simulink model "Microgrid_w_BESS"  (R2024b)
settings: Solver=VariableStepAuto  StartTime=0.0  StopTime=4  RelTol=1e-3
undefined symbols (not defined in the file or in its folder): Ion, Lithium, Ts_Control
libraries: spsParallelRLCBranchLib x8, simulink x6, spsSeriesRLCBranchLib x6, powerlib_extras x6, ee_lib x5, nesl_utility x5, slpidlib x5, spsThreePhaseVIMeasurementLib x3, spsThreePhaseSeriesRLCBranchLib x3, spsCurrentVoltageSimscapeInterfaceLib x3, eePowerMeasurement x3, spsVoltageMeasurementLib x2
(part 2 of 2)

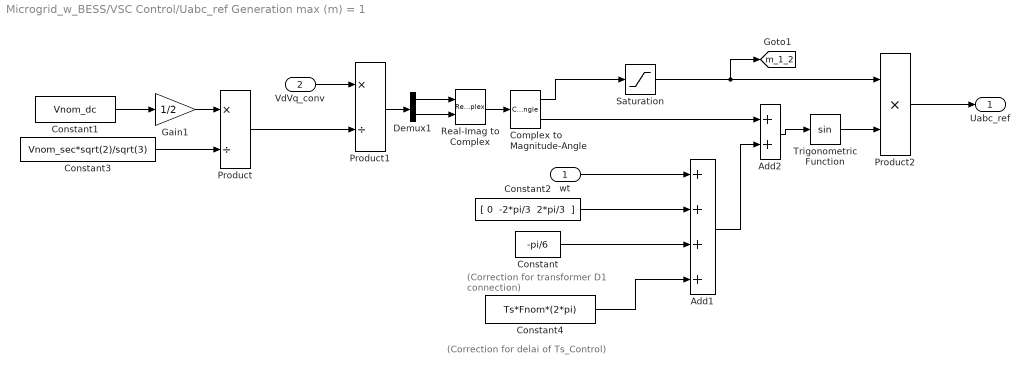
== system Microgrid_w_BESS/VSC Control/Uabc_ref Generation max (m) = 1 ==
  note: (Correction for delai of Ts_Control)
  note: (Correction for transformer
      |  D1 connection)
  wt : Inport
  VdVq_conv : Inport  Port=2
  Add1 : Sum  Inputs=++++
  Add2 : Sum
  Complex to Magnitude-Angle : ComplexToMagnitudeAngle
  Constant : Constant  Value=-pi/6
  Constant1 : Constant  Value=Vnom_dc
  Constant2 : Constant  Value="[ 0  -2*pi/3  2*pi/3  ]"
  Constant3 : Constant  Value=Vnom_sec*sqrt(2)/sqrt(3)
  Constant4 : Constant  Value=Ts*Fnom*(2*pi)
  Demux1 : Demux  Outputs=2
  Gain1 : Gain  Gain=1/2
  Product : Product  Inputs=*/  RndMeth=Zero
  Product1 : Product  Inputs=*/  RndMeth=Zero
  Product2 : Product  Inputs=**  RndMeth=Zero
  Real-Imag to Complex : RealImagToComplex
  Saturation : Saturate  UpperLimit=1  LowerLimit=0
  Trigonometric Function : Trigonometry
  Uabc_ref : Outport  VectorParamsAs1DForOutWhenUnconnected=off
  tag scope: m_1_2=global
  wires:
  Constant4/1 -> Add1/4
  wt/1 -> Add1/1
  Product2/1 -> Uabc_ref/1
  Trigonometric Function/1 -> Product2/2
  Saturation/1 -> Product2/1, [m_1_2]
  Add2/1 -> Trigonometric Function/1
  Add1/1 -> Add2/2
  Complex to Magnitude-Angle/2 -> Add2/1
  Product/1 -> Product1/2
  Constant3/1 -> Product/2
  Constant/1 -> Add1/3
  Constant2/1 -> Add1/2
  Demux1/2 -> Real-Imag to Complex/2
  Demux1/1 -> Real-Imag to Complex/1
  Real-Imag to Complex/1 -> Complex to Magnitude-Angle/1
  Gain1/1 -> Product/1
  Product1/1 -> Demux1/1
  VdVq_conv/1 -> Product1/1
  Constant1/1 -> Gain1/1
  Complex to Magnitude-Angle/1 -> Saturation/1

== system Microgrid_w_BESS/VSC Control/VDC Regulator ==
  Vdc_meas : Inport  PortDimensions=1
  Vdc_ref : Inport  Port=2  PortDimensions=1
  PI : slpidlib/PID Controller  Controller=PI  Form=Parallel  TimeDomain=Discrete-time  UseExternalTs=off  SampleTime=Ts  IntegratorMethod=Trapezoidal  FilterMethod=Forward Euler  ControllerParametersSource=internal  P=Kp_VDCreg  I=Ki_VDCreg  UseKiTs=off  D=0  UseExternalDerivativeSource=off  N=100  UseFilter=on  TunerSelectOption=Transfer Function Based (PID Tuner App)  InitialConditionSource=internal  InitialConditionForIntegrator=0  InitialConditionForFilter=0  DifferentiatorICPrevScaledInput=0  ExternalReset=none  TrackingMode=off  Kt=1  LimitOutput=on  SatLimitsSource=internal  UpperSaturationLimit=1.5  LowerSaturationLimit=-1.5  LinearizeAsGain=off  AntiWindupMode=none  Kb=1  LimitIntegrator=off  UpperIntegratorSaturationLimit=inf  LowerIntegratorSaturationLimit=-inf  POutMin=[]  POutMax=[]  IOutMin=[]  IOutMax=[]  DOutMin=[]  DOutMax=[]  NOutMin=[]  NOutMax=[]  SumOutMin=[]  SumOutMax=[]  SaturationOutMin=[]  SaturationOutMax=[]  PParamMin=[]  PParamMax=[]  IParamMin=[]  IParamMax=[]  DParamMin=[]  DParamMax=[]  NParamMin=[]  NParamMax=[]  KbParamMin=[]  KbParamMax=[]  KtParamMin=[]  KtParamMax=[]  KbOutMin=[]  KbOutMax=[]  KtOutMin=[]  KtOutMax=[]  IntegratorOutMin=[]  IntegratorOutMax=[]  FilterOutMin=[]  FilterOutMax=[]  SumI1OutMin=[]  SumI1OutMax=[]  SumI2OutMin=[]  SumI2OutMax=[]  SumI3OutMin=[]  SumI3OutMax=[]  SumI4OutMin=[]  SumI4OutMax=[]  SumDOutMin=[]  SumDOutMax=[]  DifferentiatorOutMin=[]  DifferentiatorOutMax=[]  FilterDiffOutCoefMin=[]  FilterDiffOutCoefMax=[]  ReciprocalOutMin=[]  ReciprocalOutMax=[]  SumDenOutMin=[]  SumDenOutMax=[]  SumNumOutMin=[]  SumNumOutMax=[]  DivideOutMin=[]  DivideOutMax=[]  UdiffTsProdOutMin=[]  UdiffTsProdOutMax=[]  NTsProdOutMin=[]  NTsProdOutMax=[]  UintegralTsProdOutMin=[]  UintegralTsProdOutMax=[]  UngainTsProdOutMin=[]  UngainTsProdOutMax=[]  ClampingZeroOutDataTypeStr=Inherit: Inherit via back propagation  ClampingZeroOutMin=[]  ClampingZeroOutMax=[]  FilterDenConstantOutDataTypeStr=Inherit: Inherit via back propagation  FilterDenConstantOutMin=[]  FilterDenConstantOutMax=[]  PCopyOutDataTypeStr=Inherit: Inherit via back propagation  PCopyOutMin=[]  PCopyOutMax=[]  NCopyOutDataTypeStr=Inherit: Inherit via back propagation  NCopyOutMin=[]  NCopyOutMax=[]  IntegratorContinuousStateAttributes=''  IntegratorStateMustResolveToSignalObject=off  IntegratorRTWStateStorageClass=Auto  FilterContinuousStateAttributes=''  FilterStateMustResolveToSignalObject=off  FilterRTWStateStorageClass=Auto  ParallelPVariant=InternalParameters  IdealPVariant=Disabled  IVariant=InternalParameters  DVariant=Disabled  IntegratorVariant=Discrete  SatVariant=Enabled  AWVariant=Passthrough  PCopyVariant=Disabled  TRVariant=Disabled  FdbkBlocksVariant=Forward  IdealPFdbkVariant=Disabled  SatFdbkVariant=Disabled  DerivativeFilterVariant=Disabled  NVariant=Disabled  NCopyVariant=Disabled_SignalSpec  FilterICVariant=Disabled  IntegratorICVariant=InternalICs  ExternalResetVariant=Disabled  TRSumVariant=Passthrough  SumFdbkVariant=Disabled  SumVariant=Sum_PI  TsampFilterVariant=InternalTs  TsampNgainVariant=Passthrough  TsampIntegralVariant=Disabled_SignalSpec  ExternalSaturationOutDataTypeStr=Inherit: Same as second input  DerivativeSourceVariant=Disabled  PreIntVariant=InternalPreInt
  Rtot_pu3 : Gain  Gain=1/Vnom_dc  SaturateOnIntegerOverflow=on  OutDataTypeStr=Inherit: Same as input  ParamDataTypeStr=Inherit: Same as input
  Sum : Sum  Inputs=|+-
  Id_ref : Outport  SampleTime=Ts  InitialOutput=0  VectorParamsAs1DForOutWhenUnconnected=off
  tag scope: Id_ref_2=global, Vdc_ref_2=global
  wires:
  Rtot_pu3/1 -> PI/1
  Vdc_ref/1 -> [Vdc_ref_2], Sum/2
  Vdc_meas/1 -> Sum/1
  Sum/1 -> Rtot_pu3/1
  PI/1 -> [Id_ref_2], Id_ref/1

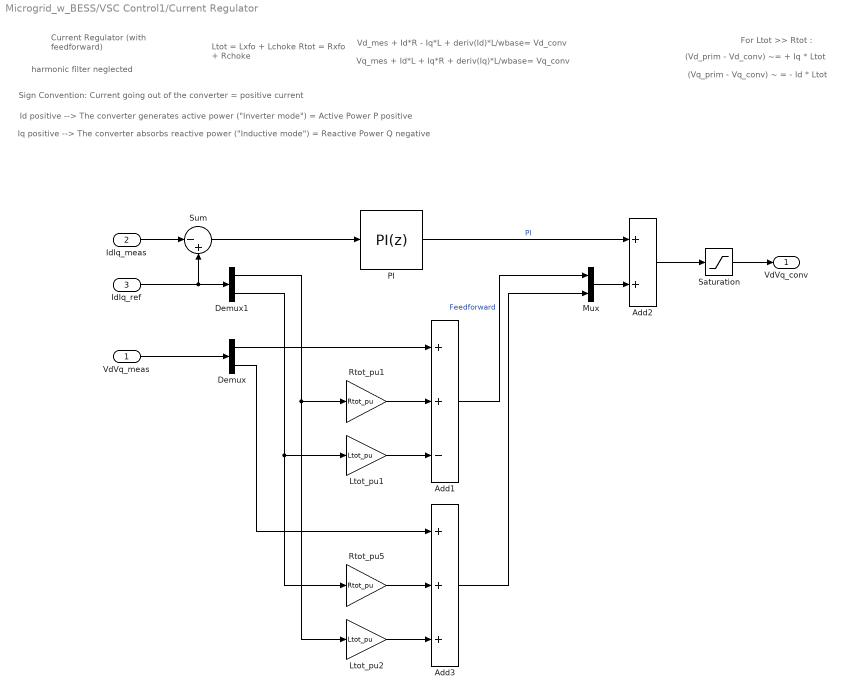
== system Microgrid_w_BESS/VSC Control1/Current Regulator ==
  note: harmonic filter neglected
  note: Vd_mes + Id*R - Iq*L + deriv(Id)*L/wbase= Vd_conv
  note: Vq_mes + Id*L + Iq*R + deriv(Iq)*L/wbase= Vq_conv
  note: Current Regulator
      | (with feedforward)
  note: Sign Convention: Current going out of the converter = positive current
  note: Iq positive --> The converter absorbs reactive power ("Inductive mode") = Reactive Power Q negative
  note: Id positive --> The converter generates active power ("Inverter mode") = Active Power P positive
  note: Ltot = Lxfo + Lchoke
      | Rtot = Rxfo + Rchoke
  note: (Vd_prim - Vd_conv) ~= + Iq * Ltot
  note: (Vq_prim - Vq_conv) ~ = - Id * Ltot
  note: For Ltot >> Rtot :
  VdVq_meas : Inport  PortDimensions=2
  IdIq_meas : Inport  Port=2  PortDimensions=2
  IdIq_ref : Inport  Port=3  PortDimensions=2
  Add1 : Sum  Inputs=++-
  Add2 : Sum
  Add3 : Sum  Inputs=+++
  Demux : Demux  Outputs=2
  Demux1 : Demux  Outputs=2
  Ltot_pu1 : Gain  Gain=Ltot_pu  SaturateOnIntegerOverflow=on  OutDataTypeStr=Inherit: Same as input  ParamDataTypeStr=Inherit: Same as input
  Ltot_pu2 : Gain  Gain=Ltot_pu  SaturateOnIntegerOverflow=on  OutDataTypeStr=Inherit: Same as input  ParamDataTypeStr=Inherit: Same as input
  Mux : Mux  Inputs=2
  PI : slpidlib/PID Controller  Controller=PI  Form=Parallel  TimeDomain=Discrete-time  UseExternalTs=off  SampleTime=Ts  IntegratorMethod=Forward Euler  FilterMethod=Forward Euler  ControllerParametersSource=internal  P=Kp_Ireg  I=Ki_Ireg  UseKiTs=off  D=0  UseExternalDerivativeSource=off  N=100  UseFilter=on  TunerSelectOption=Transfer Function Based (PID Tuner App)  InitialConditionSource=internal  InitialConditionForIntegrator=0  InitialConditionForFilter=0  DifferentiatorICPrevScaledInput=0  ExternalReset=none  TrackingMode=off  Kt=1  LimitOutput=on  SatLimitsSource=internal  UpperSaturationLimit=2  LowerSaturationLimit=-2  LinearizeAsGain=off  AntiWindupMode=none  Kb=1  LimitIntegrator=off  UpperIntegratorSaturationLimit=inf  LowerIntegratorSaturationLimit=-inf  POutMin=[]  POutMax=[]  IOutMin=[]  IOutMax=[]  DOutMin=[]  DOutMax=[]  NOutMin=[]  NOutMax=[]  SumOutMin=[]  SumOutMax=[]  SaturationOutMin=[]  SaturationOutMax=[]  PParamMin=[]  PParamMax=[]  IParamMin=[]  IParamMax=[]  DParamMin=[]  DParamMax=[]  NParamMin=[]  NParamMax=[]  KbParamMin=[]  KbParamMax=[]  KtParamMin=[]  KtParamMax=[]  KbOutMin=[]  KbOutMax=[]  KtOutMin=[]  KtOutMax=[]  IntegratorOutMin=[]  IntegratorOutMax=[]  FilterOutMin=[]  FilterOutMax=[]  SumI1OutMin=[]  SumI1OutMax=[]  SumI2OutMin=[]  SumI2OutMax=[]  SumI3OutMin=[]  SumI3OutMax=[]  SumI4OutMin=[]  SumI4OutMax=[]  SumDOutMin=[]  SumDOutMax=[]  DifferentiatorOutMin=[]  DifferentiatorOutMax=[]  FilterDiffOutCoefMin=[]  FilterDiffOutCoefMax=[]  ReciprocalOutMin=[]  ReciprocalOutMax=[]  SumDenOutMin=[]  SumDenOutMax=[]  SumNumOutMin=[]  SumNumOutMax=[]  DivideOutMin=[]  DivideOutMax=[]  UdiffTsProdOutMin=[]  UdiffTsProdOutMax=[]  NTsProdOutMin=[]  NTsProdOutMax=[]  UintegralTsProdOutMin=[]  UintegralTsProdOutMax=[]  UngainTsProdOutMin=[]  UngainTsProdOutMax=[]  ClampingZeroOutDataTypeStr=Inherit: Inherit via back propagation  ClampingZeroOutMin=[]  ClampingZeroOutMax=[]  FilterDenConstantOutDataTypeStr=Inherit: Inherit via back propagation  FilterDenConstantOutMin=[]  FilterDenConstantOutMax=[]  PCopyOutDataTypeStr=Inherit: Inherit via back propagation  PCopyOutMin=[]  PCopyOutMax=[]  NCopyOutDataTypeStr=Inherit: Inherit via back propagation  NCopyOutMin=[]  NCopyOutMax=[]  IntegratorContinuousStateAttributes=''  IntegratorStateMustResolveToSignalObject=off  IntegratorRTWStateStorageClass=Auto  FilterContinuousStateAttributes=''  FilterStateMustResolveToSignalObject=off  FilterRTWStateStorageClass=Auto  ParallelPVariant=InternalParameters  IdealPVariant=Disabled  IVariant=InternalParameters  DVariant=Disabled  IntegratorVariant=Discrete  SatVariant=Enabled  AWVariant=Passthrough  PCopyVariant=Disabled  TRVariant=Disabled  FdbkBlocksVariant=Forward  IdealPFdbkVariant=Disabled  SatFdbkVariant=Disabled  DerivativeFilterVariant=Disabled  NVariant=Disabled  NCopyVariant=Disabled_SignalSpec  FilterICVariant=Disabled  IntegratorICVariant=InternalICs  ExternalResetVariant=Disabled  TRSumVariant=Passthrough  SumFdbkVariant=Disabled  SumVariant=Sum_PI  TsampFilterVariant=InternalTs  TsampNgainVariant=Passthrough  TsampIntegralVariant=Disabled_SignalSpec  ExternalSaturationOutDataTypeStr=Inherit: Same as second input  DerivativeSourceVariant=Disabled  PreIntVariant=InternalPreInt
  Rtot_pu1 : Gain  Gain=Rtot_pu  SaturateOnIntegerOverflow=on  OutDataTypeStr=Inherit: Same as input  ParamDataTypeStr=Inherit: Same as input
  Rtot_pu5 : Gain  Gain=Rtot_pu  SaturateOnIntegerOverflow=on  OutDataTypeStr=Inherit: Same as input  ParamDataTypeStr=Inherit: Same as input
  Saturation : Saturate  UpperLimit=2  LowerLimit=-2
  Sum : Sum  Inputs=|-+
  VdVq_conv : Outport  VectorParamsAs1DForOutWhenUnconnected=off
  wires:
  Mux/1 -> Add2/2
  PI/1 -> Add2/1  "PI"
  Sum/1 -> PI/1
  IdIq_ref/1 -> Sum/2, Demux1/1
  IdIq_meas/1 -> Sum/1
  Add2/1 -> Saturation/1
  Saturation/1 -> VdVq_conv/1
  VdVq_meas/1 -> Demux/1
  Demux/1 -> Add1/1
  Rtot_pu1/1 -> Add1/2
  Demux1/1 -> Rtot_pu1/1, Ltot_pu2/1
  Ltot_pu1/1 -> Add1/3
  Demux1/2 -> Ltot_pu1/1, Rtot_pu5/1
  Rtot_pu5/1 -> Add3/2
  Ltot_pu2/1 -> Add3/3
  Add1/1 -> Mux/1  "Feedforward"
  Demux/2 -> Add3/1
  Add3/1 -> Mux/2

== system Microgrid_w_BESS/VSC Control1/Inverter ON//OFF Logic ==
  V_DC : Inport
  AND : Logic  Operator=NAND  IconShape=distinctive  AllPortsSameDT=off  OutDataTypeStr=boolean
  Compare To Constant : simulink/Logic and Bit Operations/Compare To Constant  relop=>=  const=200  OutDataTypeStr=boolean
  Constant : Constant
  Data Type Conversion : DataTypeConversion  OutDataTypeStr=double  SaturateOnIntegerOverflow=off  RndMeth=Floor
  BL : Outport
  tag scope: inv_cont_1=global
  wires:
  Constant/1 -> AND/2
  Compare To Constant/1 -> AND/1
  AND/1 -> Data Type Conversion/1
  V_DC/1 -> Compare To Constant/1
  Data Type Conversion/1 -> BL/1, [inv_cont_1]

== system Microgrid_w_BESS/VSC Control1/PLL & Measurements ==
  Vabc_prim : Inport
  Iabc_prim : Inport  Port=2
  PLL : powerlib_extras/Discrete  Control Blocks/Discrete 3-phase PLL  Fmin=45  Par_Init="[-0.57  Fnom]"  ParK=[60 1400]  Ts=Ts  AGC=off
  Selector1 : Selector  InputPortWidth=3  IndexOptions=Index vector (dialog)  Indices=[1 2]  OutputSizes=1
  Selector2 : Selector  InputPortWidth=3  IndexOptions=Index vector (dialog)  Indices=[1 2]  OutputSizes=1
  Terminator : Terminator
  V->pu : Gain  Gain=1/(Vnom_prim*sqrt(2)/sqrt(3))  SaturateOnIntegerOverflow=on  OutDataTypeStr=Inherit: Same as input  ParamDataTypeStr=Inherit: Same as input
  V->pu1 : Gain  Gain=Vnom_prim*sqrt(3)/Pnom/sqrt(2)  SaturateOnIntegerOverflow=on  OutDataTypeStr=Inherit: Same as input  ParamDataTypeStr=Inherit: Same as input
  abc_to_dq0 Transformation1 : powerlib_extras/Measurements/abc_to_dq0 Transformation
  abc_to_dq0 Transformation2 : powerlib_extras/Measurements/abc_to_dq0 Transformation
  wt : Outport  VectorParamsAs1DForOutWhenUnconnected=off
  VdVq_prim : Outport  Port=2  VectorParamsAs1DForOutWhenUnconnected=off
  IdIq_prim : Outport  Port=3  VectorParamsAs1DForOutWhenUnconnected=off
  wires:
  V->pu1/1 -> abc_to_dq0 Transformation2/1
  V->pu/1 -> PLL/1, abc_to_dq0 Transformation1/1
  abc_to_dq0 Transformation2/1 -> Selector1/1
  PLL/2 -> wt/1
  Vabc_prim/1 -> V->pu/1
  Iabc_prim/1 -> V->pu1/1
  abc_to_dq0 Transformation1/1 -> Selector2/1
  Selector2/1 -> VdVq_prim/1
  Selector1/1 -> IdIq_prim/1
  PLL/3 -> abc_to_dq0 Transformation2/2, abc_to_dq0 Transformation1/2
  PLL/1 -> Terminator/1

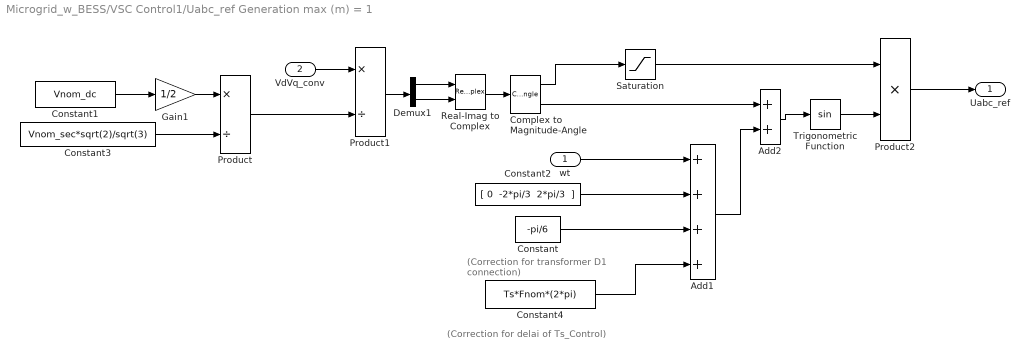
== system Microgrid_w_BESS/VSC Control1/Uabc_ref Generation max (m) = 1 ==
  note: (Correction for transformer
      |  D1 connection)
  note: (Correction for delai of Ts_Control)
  wt : Inport
  VdVq_conv : Inport  Port=2
  Add1 : Sum  Inputs=++++
  Add2 : Sum
  Complex to Magnitude-Angle : ComplexToMagnitudeAngle
  Constant : Constant  Value=-pi/6
  Constant1 : Constant  Value=Vnom_dc
  Constant2 : Constant  Value="[ 0  -2*pi/3  2*pi/3  ]"
  Constant3 : Constant  Value=Vnom_sec*sqrt(2)/sqrt(3)
  Constant4 : Constant  Value=Ts*Fnom*(2*pi)
  Demux1 : Demux  Outputs=2
  Gain1 : Gain  Gain=1/2
  Product : Product  Inputs=*/  RndMeth=Zero
  Product1 : Product  Inputs=*/  RndMeth=Zero
  Product2 : Product  Inputs=**  RndMeth=Zero
  Real-Imag to Complex : RealImagToComplex
  Saturation : Saturate  UpperLimit=1  LowerLimit=0
  Trigonometric Function : Trigonometry
  Uabc_ref : Outport  VectorParamsAs1DForOutWhenUnconnected=off
  wires:
  Complex to Magnitude-Angle/1 -> Saturation/1
  Constant1/1 -> Gain1/1
  VdVq_conv/1 -> Product1/1
  Product1/1 -> Demux1/1
  Gain1/1 -> Product/1
  Real-Imag to Complex/1 -> Complex to Magnitude-Angle/1
  Demux1/1 -> Real-Imag to Complex/1
  Demux1/2 -> Real-Imag to Complex/2
  Constant2/1 -> Add1/2
  Constant/1 -> Add1/3
  Constant3/1 -> Product/2
  Product/1 -> Product1/2
  Complex to Magnitude-Angle/2 -> Add2/1
  Add1/1 -> Add2/2
  Add2/1 -> Trigonometric Function/1
  Saturation/1 -> Product2/1
  Trigonometric Function/1 -> Product2/2
  Product2/1 -> Uabc_ref/1
  wt/1 -> Add1/1
  Constant4/1 -> Add1/4

== system Microgrid_w_BESS/VSC Control1/VDC Regulator ==
  Vdc_meas : Inport  PortDimensions=1
  Vdc_ref : Inport  Port=2  PortDimensions=1
  PI : slpidlib/PID Controller  Controller=PI  Form=Parallel  TimeDomain=Discrete-time  UseExternalTs=off  SampleTime=Ts  IntegratorMethod=Trapezoidal  FilterMethod=Forward Euler  ControllerParametersSource=internal  P=Kp_VDCreg  I=Ki_VDCreg  UseKiTs=off  D=0  UseExternalDerivativeSource=off  N=100  UseFilter=on  TunerSelectOption=Transfer Function Based (PID Tuner App)  InitialConditionSource=internal  InitialConditionForIntegrator=0  InitialConditionForFilter=0  DifferentiatorICPrevScaledInput=0  ExternalReset=none  TrackingMode=off  Kt=1  LimitOutput=on  SatLimitsSource=internal  UpperSaturationLimit=1.5  LowerSaturationLimit=-1.5  LinearizeAsGain=off  AntiWindupMode=none  Kb=1  LimitIntegrator=off  UpperIntegratorSaturationLimit=inf  LowerIntegratorSaturationLimit=-inf  POutMin=[]  POutMax=[]  IOutMin=[]  IOutMax=[]  DOutMin=[]  DOutMax=[]  NOutMin=[]  NOutMax=[]  SumOutMin=[]  SumOutMax=[]  SaturationOutMin=[]  SaturationOutMax=[]  PParamMin=[]  PParamMax=[]  IParamMin=[]  IParamMax=[]  DParamMin=[]  DParamMax=[]  NParamMin=[]  NParamMax=[]  KbParamMin=[]  KbParamMax=[]  KtParamMin=[]  KtParamMax=[]  KbOutMin=[]  KbOutMax=[]  KtOutMin=[]  KtOutMax=[]  IntegratorOutMin=[]  IntegratorOutMax=[]  FilterOutMin=[]  FilterOutMax=[]  SumI1OutMin=[]  SumI1OutMax=[]  SumI2OutMin=[]  SumI2OutMax=[]  SumI3OutMin=[]  SumI3OutMax=[]  SumI4OutMin=[]  SumI4OutMax=[]  SumDOutMin=[]  SumDOutMax=[]  DifferentiatorOutMin=[]  DifferentiatorOutMax=[]  FilterDiffOutCoefMin=[]  FilterDiffOutCoefMax=[]  ReciprocalOutMin=[]  ReciprocalOutMax=[]  SumDenOutMin=[]  SumDenOutMax=[]  SumNumOutMin=[]  SumNumOutMax=[]  DivideOutMin=[]  DivideOutMax=[]  UdiffTsProdOutMin=[]  UdiffTsProdOutMax=[]  NTsProdOutMin=[]  NTsProdOutMax=[]  UintegralTsProdOutMin=[]  UintegralTsProdOutMax=[]  UngainTsProdOutMin=[]  UngainTsProdOutMax=[]  ClampingZeroOutDataTypeStr=Inherit: Inherit via back propagation  ClampingZeroOutMin=[]  ClampingZeroOutMax=[]  FilterDenConstantOutDataTypeStr=Inherit: Inherit via back propagation  FilterDenConstantOutMin=[]  FilterDenConstantOutMax=[]  PCopyOutDataTypeStr=Inherit: Inherit via back propagation  PCopyOutMin=[]  PCopyOutMax=[]  NCopyOutDataTypeStr=Inherit: Inherit via back propagation  NCopyOutMin=[]  NCopyOutMax=[]  IntegratorContinuousStateAttributes=''  IntegratorStateMustResolveToSignalObject=off  IntegratorRTWStateStorageClass=Auto  FilterContinuousStateAttributes=''  FilterStateMustResolveToSignalObject=off  FilterRTWStateStorageClass=Auto  ParallelPVariant=InternalParameters  IdealPVariant=Disabled  IVariant=InternalParameters  DVariant=Disabled  IntegratorVariant=Discrete  SatVariant=Enabled  AWVariant=Passthrough  PCopyVariant=Disabled  TRVariant=Disabled  FdbkBlocksVariant=Forward  IdealPFdbkVariant=Disabled  SatFdbkVariant=Disabled  DerivativeFilterVariant=Disabled  NVariant=Disabled  NCopyVariant=Disabled_SignalSpec  FilterICVariant=Disabled  IntegratorICVariant=InternalICs  ExternalResetVariant=Disabled  TRSumVariant=Passthrough  SumFdbkVariant=Disabled  SumVariant=Sum_PI  TsampFilterVariant=InternalTs  TsampNgainVariant=Passthrough  TsampIntegralVariant=Disabled_SignalSpec  ExternalSaturationOutDataTypeStr=Inherit: Same as second input  DerivativeSourceVariant=Disabled  PreIntVariant=InternalPreInt
  Rtot_pu3 : Gain  Gain=1/Vnom_dc  SaturateOnIntegerOverflow=on  OutDataTypeStr=Inherit: Same as input  ParamDataTypeStr=Inherit: Same as input
  Sum : Sum  Inputs=|+-
  Id_ref : Outport  SampleTime=Ts  InitialOutput=0  VectorParamsAs1DForOutWhenUnconnected=off
  wires:
  PI/1 -> Id_ref/1
  Sum/1 -> Rtot_pu3/1
  Vdc_meas/1 -> Sum/1
  Vdc_ref/1 -> Sum/2
  Rtot_pu3/1 -> PI/1

== system Microgrid_w_BESS/BESS/BATT chg-dshg logic1/Unused ==
  Charging : Constant  Commented=on
  MATLAB Function : MATLAB Function  Commented=on  TreatAsAtomicUnit=on
  MATLAB Function1 : MATLAB Function  Commented=on  TreatAsAtomicUnit=on
  MATLAB Function2 : MATLAB Function  Commented=on  TreatAsAtomicUnit=on
  MATLAB Function7 : MATLAB Function  Commented=on  TreatAsAtomicUnit=on
  MATLAB Function8 : MATLAB Function  Commented=on  TreatAsAtomicUnit=on
  Manual Switch : ManualSwitch  Commented=on  CurrentSetting=0
  discharging : Constant  Commented=on  Value=0
  Out1 : Outport
  wires:
  Manual Switch/1 -> Out1/1
  Charging/1 -> Manual Switch/2
  discharging/1 -> Manual Switch/1

== matlab function Microgrid_w_BESS/BESS/BATT chg-dshg logic1/Unused/MATLAB Function7 ==
  data: Vdc input; D output; Vbatt input; I_batt_meas input; I_batt_ref_mag input; Ts input
function D = controller_discharging(Vdc, Vbatt, I_batt_meas, I_batt_ref_mag, Ts)
%#codegen
% Limits
Imax_discharge = -50;
% PI gains for discharging (tuned for damping)
Kp = 0.3; % Increased for quicker response
Ki = 0.9; % Moderate integral action
Kd = 0.001; % Small derivative term for damping
persistent integral_error prev_error
if isempty(integral_error)
    integral_error = 0;
    prev_error = 0;
end
% Current reference
I_batt_ref = -I_batt_ref_mag;
% Clamp current reference
I_batt_ref = max(I_batt_ref, Imax_discharge);
% PI control with derivative and anti-windup
error = I_batt_ref - I_batt_meas;
integral_error = max(min(integral_error + error * Ts, 200), -200); % Anti-windup
derivative = (error - prev_error) / Ts; % Derivative term
PI_output = Kp * error + Ki * integral_error + Kd * derivative;
prev_error = error;
% Base duty calculation (boost mode)
D_base = 1 - Vbatt / Vdc;
% Total duty
D = D_base + PI_output;
D = max(min(D, 0.95), 0.05); % Limit duty cycle
% Debugging
assignin('base', 'I_batt_ref', I_batt_ref);
assignin('base', 'I_batt_meas', I_batt_meas);
assignin('base', 'integral_error', integral_error);
assignin('base', 'D', D);
end

== matlab function Microgrid_w_BESS/Scopes/SoC/MATLAB Function1 ==
  settings: updateMethod=DISCRETE
  data: I_batt input; SoC output; V_batt input; initial_SOC input; Q_nom input; time_scale input; Ts input
function SoC = soc_estimation_with_voltage(I_batt, V_batt, initial_SOC, Q_nom, time_scale, Ts)
%#codegen
% Persistent integrator state
persistent integral_charge
if isempty(integral_charge)
    integral_charge = 0;
end
% Time-scaled charge integration (Ah)
delta_charge = (I_batt * Ts) / 3600; % Charge in Ah per step
integral_charge = integral_charge + delta_charge * time_scale; % Scale for 24h in 4s
% Coulomb-based SoC (no upper clamp to allow proper discharge)
SoC_coulomb = initial_SOC - (integral_charge / Q_nom); % Direct use of Q_nom
% Voltage-based correction
V_corr = V_batt + I_batt * 0.1; % Compensate for voltage drop (R_int = 0.1 Ohm)
SoC_voltage = max(0, min(1, (V_corr - 300) / 150)); % Adjusted range, clamped
% Weighted average with minimal voltage influence
SoC = 0.98 * SoC_coulomb + 0.02 * SoC_voltage; % Rely heavily on coulomb
% Apply final limits
SoC = max(0, min(0.9, SoC)); % Clamp between 0 and 90%
% Debugging (log to Workspace)
assignin('base', 'integral_charge', integral_charge);
assignin('base', 'delta_charge', delta_charge);
assignin('base', 'I_batt', I_batt);
end

== matlab function Microgrid_w_BESS/BESS/BATT chg-dshg logic1/Unused/MATLAB Function8 ==
  data: Vdc input; D output; Vbatt input; I_batt_meas input; I_batt_ref_mag input
% controller_charging.m
% PI control for bidirectional DC-DC converter in charging (buck) mode
 
function D = controller_charging(Vdc, Vbatt, I_batt_meas, I_batt_ref_mag)
%#codegen
 
% Limits
Imax_charge = 50;
 
% PI gains for charging
Kp = 0.01;
Ki = 0.05;
persistent integral_error
if isempty(integral_error)
    integral_error = 0;
end
 
% Current reference
I_batt_ref = I_batt_ref_mag;
 
% Clamp current reference
I_batt_ref = min(I_batt_ref, Imax_charge);
 
% PI control
error = I_batt_ref - I_batt_meas;
dt = 1e-4; % Match to 10 kHz switching
integral_error = integral_error + error * dt; % No anti-windup for simplicity
PI_output = Kp * error + Ki * integral_error;
 
% Base duty calculation (buck mode)
D_base = Vbatt / Vdc;
 
% Total duty
D = D_base + PI_output;
D = max(min(D, 0.9), 0.05); % Limit duty cycle
 
end

== matlab function Microgrid_w_BESS/BESS/BATT chg-dshg logic1/Unused/MATLAB Function1 ==
  settings: updateMethod=DISCRETE
  data: Vdc input; Vbatt input; I_batt_meas input; P_pv input; P_load input; SoC input; D output
% =========================================================================
% Unified PI controller + supervisory logic for a bidirectional DC-DC BESS
% Outputs duty-ratio D directly
%
% Inputs  (all scalars, sampled each control step – e.g. 100 µs)
%   Vdc         – DC-link voltage           [V]
%   Vbatt       – battery terminal voltage  [V]
%   I_batt_meas – measured battery current  [A]  (+ve = charging)
%   P_pv        – instantaneous PV power    [W]  (+ve = generation)
%   P_load      – instantaneous load power  [W]  (+ve = consumption)
%   SoC         – battery state-of-charge   [0…1]
%
% Output
%   D           – duty cycle for the half-bridge (0.05…0.95)
%
% Author: 2025-06-19
% =========================================================================
function D = bidirectional_controller( ...
                  Vdc, Vbatt, I_batt_meas, P_pv, P_load, SoC) %#codegen
% ---------- user-tunable limits ------------------------------------------
Imax_charge   =  50;      % [A]  charge current limit  (+)
Imax_discharge= -50;      % [A]  discharge limit       (-)
SoC_min       = 0.10;     % 10 %: stop discharging below this
P_dead        = 50;       % [W]  dead-band to avoid chattering
% -------------------------------------------------------------------------

% ---------- supervisory layer (decide charge / discharge / idle) ---------
P_net = P_pv - P_load;    % +ve ⇒ surplus PV power available

if  (P_net >  P_dead)          && (SoC < 1)        % charge allowed
    mode = 0;                                       % 0 = charge
    I_batt_ref_mag =  P_net / max(Vbatt,1e-3);      % >0
elseif (P_net < -P_dead)         && (SoC > SoC_min) % discharge allowed
    mode = 1;                                       % 1 = discharge
    I_batt_ref_mag = -P_net / max(Vbatt,1e-3);      % >0
else                                                 % dead-band / SoC lim
    mode = 2;                                       % 2 = idle
    I_batt_ref_mag = 0;
end

% ---------- inner PI current loop ----------------------------------------
% Persistent integrator state
persistent integral_error
if isempty(integral_error); integral_error = 0; end

% Adjust sign of reference
if mode == 0
    I_batt_ref =  I_batt_ref_mag;       % charge (+)
elseif mode == 1
    I_batt_ref = -I_batt_ref_mag;       % discharge (-)
else
    I_batt_ref = 0;                     % idle
end

% Clamp current reference to hard limits
I_batt_ref = max(min(I_batt_ref, Imax_charge), Imax_discharge);

% PI gains (tune to taste)
Kp = 0.9;
Ki = 0.5;

% PI computation
error = I_batt_ref - I_batt_meas;
dt    = 1e-4;                           % 100 µs sample
integral_error = integral_error + error*dt;
PI_output      = Kp*error + Ki*integral_error;

% ---------- duty-ratio synthesis -----------------------------------------
if     mode == 0          % Buck (charge)
    D_base =  Vbatt / Vdc;
elseif mode == 1          % Boost (discharge)
    D_base = 1 - Vbatt / Vdc;
else                      % idle → open-circuit
    D_base = 0;
end

D = D_base + PI_output;
D = min(max(D,0.05),0.95);   % PWM guard-rails
end

== matlab function Microgrid_w_BESS/BESS/BATT chg-dshg logic1/MATLAB Function1 ==
  settings: updateMethod=DISCRETE
  data: mode input; D output; V_batt input; V_dc input; I_meas input; I_ref input
function D = compute_duty_cycle(mode, V_batt, V_dc, I_meas, I_ref)
% compute_duty_cycle - Calculates duty cycle for bidirectional DC-DC converter
% using a PI controller to regulate battery current.
%
% Inputs:
%   mode   - 1 = charging, 0 = discharging
%   V_batt - battery voltage [V]
%   V_dc   - DC bus voltage [V]
%   I_meas - measured battery current [A]
%   I_ref  - reference battery current [A]
%
% Output:
%   D      - duty cycle (0.05 to 0.95)

    % --- PI Controller Gains ---
    Kp = 0.005;     % Proportional gain
    Ki = 50;        % Integral gain
    Ts = 1e-4;      % Sampling time [s]

    % --- Controller Output Limits (u) ---
    u_min = 5;      % Minimum control output voltage
    u_max = 100;    % Maximum control output voltage

    % --- Persistent Integral Term ---
    persistent integral_err;
    if isempty(integral_err)
        integral_err = 0;
    end

    % --- Current Error ---
    err = I_ref - I_meas;

    % --- Proportional Term ---
    P_term = Kp * err;

    % --- Integral Term (Anti-Windup Logic) ---
    u_unclamped = P_term + Ki * integral_err;

    % Apply clamping
    u = min(max(u_unclamped, u_min), u_max);

    % Update integrator only if not saturated
    if u == u_unclamped
        integral_err = integral_err + err * Ts;
    end

    % --- Duty Cycle Calculation Based on Mode ---
    if mode == 1
        % Charging → Buck mode
        D = u / V_dc;
    elseif mode == 0
        % Discharging → Boost mode
        D = 1 - (V_batt / u);
    else
        D = 0.5; % fallback value
    end

    % --- Clamp Final Duty Cycle Output ---
    D = min(max(D, 0.05), 0.95);
end

== matlab function Microgrid_w_BESS/BESS/BATT chg-dshg logic1/Unused/MATLAB Function2 ==
  data: P_bess input; D output; V_batt input; V_dc input; efficiency input; max_power input
% p_bess_to_duty_cycle.m
% Convert BESS power command (P_bess) to duty cycle (D) for bidirectional boost converter

function D = p_bess_to_duty_cycle(P_bess, V_batt, V_dc, efficiency, max_power)
    % Inputs:
    %   P_bess: BESS power command (kW, positive for discharge, negative for charge)
    %   V_batt: BESS voltage (V)
    %   V_dc: DC-link voltage at PCC (V)
    %   efficiency: Converter efficiency (0 to 1)
    %   max_power: Max BESS power (kW)
    % Output:
    %   D: Duty cycle (0 to 1) for converter PWM control

    % Convert P_bess to watts
    P_bess_w = P_bess * 1000;

    % Limit P_bess to max_power
    P_bess_w = max(-max_power * 1000, min(max_power * 1000, P_bess_w));

    if P_bess_w > 0
        % Discharge (Boost Mode)
        % Calculate battery current: I_batt = P_bess / (V_batt * efficiency)
        I_batt = P_bess_w / (V_batt * efficiency);
        % Boost mode duty cycle: D = 1 - V_batt / V_dc
        D = 1 - V_batt / V_dc;
        % Adjust D for current control (simplified linear approximation)
        % Ensure D stays within valid range
        D = max(0, min(1, D));
    elseif P_bess_w < 0
        % Charge (Buck Mode)
        % Calculate battery current: I_batt = -P_bess * efficiency / V_batt
        I_batt = -P_bess_w * efficiency / V_batt;
        % Buck mode duty cycle: D = V_batt / V_dc
        D = V_batt / V_dc;
        % Adjust D for current control (simplified linear approximation)
        % Ensure D stays within valid range
        D = max(0, min(1, D));
    else
        % No power flow
        D = 0;
    end
end

== matlab function Microgrid_w_BESS/BESS/BATT chg-dshg logic1/Unused/MATLAB Function ==
  settings: updateMethod=DISCRETE
  data: Vdc input; Vbatt input; I_batt_meas input; I_batt_ref_mag input; mode input; D output; Ts input
function D = bidirectional_controller(Vdc, Vbatt, I_batt_meas, I_batt_ref_mag, mode, Ts)
%#codegen

% Limits
Imax_charge = 50;
Imax_discharge = -50;

% PI gains (adjusted for better response)
Kp = 0.3;
Ki = 1.5;
persistent integral_error
if isempty(integral_error)
    integral_error = 0;
end

% Adjust reference sign based on mode
if mode == 0
    I_batt_ref = I_batt_ref_mag;      % Charging
elseif mode == 1
    I_batt_ref = -I_batt_ref_mag;     % Discharging
else
    I_batt_ref = 0;
end

% Clamp current reference
I_batt_ref = max(min(I_batt_ref, Imax_charge), Imax_discharge);

% PI control with integral clamping
error = I_batt_ref - I_batt_meas;
integral_error = max(min(integral_error + error * Ts, 100), -100); % Clamp integral
PI_output = Kp * error + Ki * integral_error;

% Base duty calculation
if mode == 0
    D_base = Vbatt / Vdc;             % Buck mode
elseif mode == 1
    D_base = 1 - Vbatt / Vdc;         % Boost mode
else
    D_base = 0;
end

% Total duty
D = D_base + PI_output;
D = min(max(D, 0.05), 0.95);
end

== matlab function Microgrid_w_BESS/Subsystem/MPPT1/MATLAB Function1 ==
  data: ipv input; Vmpp output; vpv input
function Vmpp = mppt_inccond(ipv, vpv)
    % Incremental Conductance MPPT to output Vmpp
    % Inputs:
    %   ipv - PV current (A)
    %   vpv - PV voltage (V)
    % Output:
    %   Vmpp - Maximum power point voltage (V)

    % Persistent variables to store previous states
    persistent I_prev V_prev Vpv_ref_prev

    % Initialize persistent variables
    if isempty(I_prev)
        I_prev = ipv;
        V_prev = vpv;
        Vpv_ref_prev = 364.5;     % Initial guess near Vmpp
    end

    % Parameters
    delta_Vpv = 1.5;           % Step size for Vpv_ref adjustment
    tol = 1e-4;                % MPP detection tolerance
    v_min = 5;                 % Minimum voltage threshold

    % Handle invalid inputs
    if isnan(ipv) || isnan(vpv) || vpv < v_min
        Vmpp = Vpv_ref_prev;
        return;
    end

    % Incremental Conductance Algorithm
    delta_I = ipv - I_prev;
    delta_V = vpv - V_prev;

    if abs(delta_V) < 1e-4
        if delta_I > 1e-3
            Vpv_ref = Vpv_ref_prev + delta_Vpv;
        elseif delta_I < -1e-3
            Vpv_ref = Vpv_ref_prev - delta_Vpv;
        else
            Vpv_ref = Vpv_ref_prev;
        end
    else
        inst_cond = ipv / vpv;
        inc_cond = delta_I / delta_V;

        if abs(inc_cond + inst_cond) < tol
            Vpv_ref = Vpv_ref_prev;
        elseif inc_cond > -inst_cond
            Vpv_ref = Vpv_ref_prev + delta_Vpv;
        else
            Vpv_ref = Vpv_ref_prev - delta_Vpv;
        end
    end

    % Clamp Vpv_ref to safe range
    Vpv_ref = max(364.5, max(150, Vpv_ref));

    % Output Vmpp
    Vmpp = Vpv_ref;

    % Update states
    I_prev = ipv;
    V_prev = vpv;
    Vpv_ref_prev = Vpv_ref;
end

== matlab function Microgrid_w_BESS/BESS/BATT chg-dshg logic1/MATLAB Function3 ==
  data: P_bess input; mode output; Vbatt input; Vdc input; I_batt_ref_mag output
function [mode, I_batt_ref_mag] = mode_selector(P_bess, Vbatt, Vdc)
    % Convert power to current reference
    I_batt_ref = P_bess / Vbatt; % Approximate current (ignoring losses for simplicity)
    
    if P_bess > 0
        mode = 0; % Discharging
        I_batt_ref_mag = abs(I_batt_ref);
    elseif P_bess < 0
        mode = 1; % Charging
        I_batt_ref_mag = abs(I_batt_ref);
    else
        mode = 1; % Default to charging or idle
        I_batt_ref_mag = 0;
    end
end

== matlab function Microgrid_w_BESS/BESS/BATT chg-dshg logic1/MATLAB Function4 ==
  data: P_load input; P_pv input; P_bess output; SOC input; threshold input; max_power input; SOC_min input; SOC_max input; efficiency input; disconnect_signal input; tolerance input; disconnect_flag output; dynamic_tariff input
function [P_bess, disconnect_flag] = peak_shaving_logic(P_load, P_pv, SOC, threshold, max_power, SOC_min, SOC_max, efficiency, disconnect_signal, tolerance, dynamic_tariff)
    % Peak shaving and tariff-based control logic with BESS disconnection
    % Inputs:
    %   P_load: Load power at PCC (kW)
    %   P_pv: PV generation power (kW)
    %   SOC: BESS state of charge (0 to 1)
    %   threshold: Grid power limit (kW)
    %   max_power: Max BESS power (kW)
    %   SOC_min, SOC_max: SOC limits
    %   efficiency: Round-trip efficiency
    %   disconnect_signal: External signal (1 = disconnect, 0 = connect)
    %   tolerance: Load threshold tolerance (kW) for disconnection
    %   dynamic_tariff: Current electricity tariff (currency/kWh)
    % Outputs:
    %   P_bess: BESS power (kW, positive = discharge, negative = charge)
    %   disconnect_flag: 1 = disconnect BESS, 0 = connect

    % Initialize outputs
    P_bess = 0;
    disconnect_flag = 0;

    % Net load after PV generation
    P_net = P_load - P_pv;

    % Check if BESS should be disconnected
    if disconnect_signal == 1 || abs(P_net - threshold) < tolerance || SOC <= SOC_min || SOC >= SOC_max
        P_bess = 0; % No power flow
        disconnect_flag = 1; % Signal disconnection
    else
        % Tariff-based decision threshold (e.g., charge if tariff < 0.1, discharge if > 0.2)
        if dynamic_tariff < 20 && SOC < SOC_max && P_net < threshold
            % Charge during low tariff if excess PV or low load
            P_bess = -min(threshold - P_net, max_power) / efficiency;
        elseif dynamic_tariff > 20 && SOC > SOC_min && P_net > threshold
            % Discharge during high tariff if load exceeds threshold
            P_bess = min(P_net - threshold, max_power) * efficiency;
        elseif P_net > threshold && SOC > SOC_min
            % Discharge during peak load if SOC allows
            P_bess = min(P_net - threshold, max_power) * efficiency;
        elseif P_net < threshold && SOC < SOC_max
            % Charge during off-peak if SOC allows
            P_bess = -min(threshold - P_net, max_power) / efficiency;
        else
            % No action (already set P_bess = 0)
            disconnect_flag = 1; % Disconnect if no action needed
        end
    end

    % Debugging
    assignin('base', 'P_bess', P_bess);
    assignin('base', 'disconnect_flag', disconnect_flag);
    assignin('base', 'P_net', P_net);
    assignin('base', 'SOC', SOC);
end

== matlab function Microgrid_w_BESS/Scopes/SoC/MATLAB Function ==
  settings: updateMethod=DISCRETE
  data: Q_capacity input; SOC output; SOC_initial input; I input; time input
function SOC = calculateSOC(Q_capacity, SOC_initial, I, time)
    % calculateSOC - Calculates State of Charge (SOC) based on current integration
    % Inputs:
    %   Q_capacity - Battery capacity in Ah
    %   SOC_initial - Initial SOC in percentage
    %   I - Current data array (in A)
    %   time - Time vector (in s)
    % Output:
    %   SOC - Array of SOC values over time (in percentage)

    % Initialize SOC array
    SOC = zeros(size(I));
    SOC(1) = SOC_initial; % Set initial SOC

    % SOC calculation with variable time steps
    for t = 2:length(I)
        % Time difference (s)
        dt = time(t) - time(t-1);
        % Charge transferred (Ah) = Current (A) * Time (h)
        dQ = I(t) * (dt / 3600); % Charge increment (Ah)
        
        % Update SOC based on net charge
        SOC(t) = SOC(t-1) - (dQ / Q_capacity) * 100; % Decrease SOC on discharge, increase on charge
        
        % Bound SOC between 0% and 100%
        SOC(t) = max(0, min(100, SOC(t)));
    end
end

== matlab function Microgrid_w_BESS/BESS/BATT chg-dshg logic1/MATLAB Function5 ==
  data: Vdc input; D output; Vbatt input; I_batt_meas input; I_batt_ref_mag input; Ts input
function D = controller_discharging(Vdc, Vbatt, I_batt_meas, I_batt_ref_mag, Ts)
%#codegen
% Limits
Imax_discharge = -50; % Maximum discharge current (negative)

% PID gains for discharging (tuned for stability)
Kp = 0.3; % Proportional gain
Ki = 0.7; % Integral gain
Kd = 0.002; % Derivative gain
persistent integral_error prev_error prev_I_batt_meas
if isempty(integral_error)
    integral_error = 0;
    prev_error = 0;
    prev_I_batt_meas = 0;
end

% Current reference
I_batt_ref = -I_batt_ref_mag; % Discharge reference (e.g., -50 A based on I_batt_ref_mag)
I_batt_ref = min(I_batt_ref, Imax_discharge); % Clamp to maximum discharge

% PID control with derivative and anti-windup
error = I_batt_ref - I_batt_meas;
integral_error = max(min(integral_error + error * Ts, 200), -200); % Anti-windup
derivative = (error - prev_error) / Ts; % Standard derivative term
PI_output = Kp * error + Ki * integral_error + Kd * derivative;
prev_error = error;
prev_I_batt_meas = I_batt_meas;

% Base duty calculation (boost mode)
D_base = 1 - Vbatt / Vdc;

% Total duty with adjusted limits
D = D_base + PI_output;
D = max(min(D, 0.9), 0.1); % Practical limits for boost converter

% Debugging
assignin('base', 'I_batt_ref', I_batt_ref);
assignin('base', 'I_batt_meas', I_batt_meas);
assignin('base', 'integral_error', integral_error);
assignin('base', 'D', D);
end

== matlab function Microgrid_w_BESS/BESS/BATT chg-dshg logic1/MATLAB Function6 ==
  data: Vdc input; D output; Vbatt input; I_batt_meas input; I_batt_ref_mag input; Ts input
function D = controller_charging(Vdc, Vbatt, I_batt_meas, I_batt_ref_mag, Ts)
%#codegen
% Limits
Imax_charge = 50;
Vbatt_ref = 410; % Target voltage during charging (e.g., max voltage)
R_eq = 0.1; % Equivalent resistance (battery R_int)

% PI gains for charging
Kp_i = 0.5; % Proportional gain for current
Ki_i = 1.0; % Integral gain for current
Kp_v = 0.05; % Voltage proportional gain
Ki_v = 0.5;  % Adjusted integral gain for voltage (previously 0.1)
persistent integral_error_i integral_error_v
if isempty(integral_error_i)
    integral_error_i = 0;
    integral_error_v = 0;
end

% Current reference
I_batt_ref = I_batt_ref_mag; % Positive (e.g., 50 A)
I_batt_ref = min(I_batt_ref, Imax_charge); % Clamp to 50 A

% Voltage regulation (outer loop)
error_v = Vbatt_ref - Vbatt; % Error as difference from target voltage
integral_error_v = max(min(integral_error_v + error_v * Ts, 50), -50); % Anti-windup
I_batt_ref_adj = I_batt_ref + Kp_v * error_v + Ki_v * integral_error_v; % Increase current if Vbatt < Vbatt_ref
I_batt_ref_adj = max(min(I_batt_ref_adj, Imax_charge), 0); % Limit adjusted current

% Current control (inner loop)
error_i = I_batt_ref_adj - I_batt_meas; % Positive if I_batt_meas < I_batt_ref
integral_error_i = max(min(integral_error_i + error_i * Ts, 200), -200); % Anti-windup
PI_output = Kp_i * error_i + Ki_i * integral_error_i;

% Feedforward duty calculation (buck mode)
if Vdc < 1e-6 % Safety check for near-zero Vdc
    D_base = 0.5;
else
    D_base = (Vbatt + I_batt_ref * R_eq) / Vdc; % Feedforward term
end
if Vbatt < 350 || Vbatt > 500
    D_base = 0.5; % Fallback for incorrect Vbatt
end

% Total duty
D = D_base + PI_output;
D = max(min(D, 0.9), 0.1); % Practical limits for buck converter

% Debugging
assignin('base', 'I_batt_ref', I_batt_ref);
assignin('base', 'I_batt_ref_adj', I_batt_ref_adj);
assignin('base', 'I_batt_meas', I_batt_meas);
assignin('base', 'error_i', error_i);
assignin('base', 'error_v', error_v);
assignin('base', 'integral_error_i', integral_error_i);
assignin('base', 'integral_error_v', integral_error_v);
assignin('base', 'PI_output', PI_output);
assignin('base', 'D_base', D_base);
assignin('base', 'D', D);
assignin('base', 'Vbatt', Vbatt);
assignin('base', 'Vdc', Vdc);
end
